simulink model "DegradationParameterMotor"  (R2021a)
settings: Solver=VariableStepAuto  StartTime=0.0  StopTime=10.0  RelTol=1e-3
values from neighbouring files (symbols this model uses):
  mot_P_Fe_Nom_adjustment = 0.5    [Run_GeneratorRectifierBoostConverterInverterMotorModel.m]    (also in Run_InverterMotorModel.m)
  mot_R_s_adjustment = 0.5    [Run_GeneratorRectifierBoostConverterInverterMotorModel.m]    (also in Run_InverterMotorModel.m)
  mot_S_nom_adjustment = 0.5    [Run_GeneratorRectifierBoostConverterInverterMotorModel.m]    (also in Run_InverterMotorModel.m)
undefined symbols (not defined in the file or in its folder): mot_flux_m_adjustment
libraries: Lib_EMTAT x5
settings Model: Creator=sfaulk  LastModifiedBy=mebell

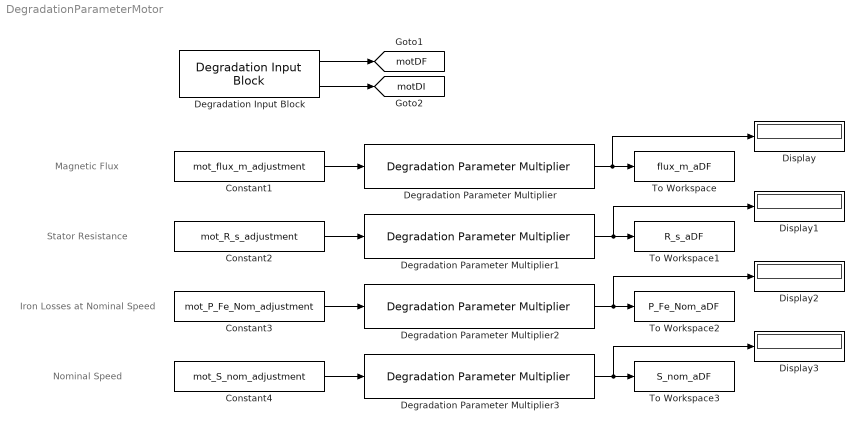
== system DegradationParameterMotor ==
  note: Stator Resistance
  note: Magnetic Flux
  note: Iron Losses at Nominal Speed
  note: Nominal Speed
  Constant1 : Constant  Value=mot_flux_m_adjustment
  Constant2 : Constant  Value=mot_R_s_adjustment
  Constant3 : Constant  Value=mot_P_Fe_Nom_adjustment
  Constant4 : Constant  Value=mot_S_nom_adjustment
  Degradation Input Block : Lib_EMTAT/Components/Physics-Based/Degradation Input Block  SystemSampleTime=-1  VariantActivationTime=update diagram  Latency=0  AutoFrameSizeCalculation=off
      settings: SourceProductName=EMTAT
  Degradation Parameter Multiplier{,1..3} (4 alike) : Lib_EMTAT/Components/Physics-Based/Degradation Parameter Multiplier  SystemSampleTime=-1  VariantActivationTime=update diagram  Latency=0  AutoFrameSizeCalculation=off
      settings: SourceProductName=EMTAT
  Display{,1..3} (4 alike) : Display
  To Workspace : ToWorkspace  VariableName=flux_m_aDF  SaveFormat=Timeseries  SampleTime=-1
      settings: Save2DSignal=2-D array (concatenate along first dimension)
  To Workspace1 : ToWorkspace  VariableName=R_s_aDF  SaveFormat=Timeseries  SampleTime=-1
      settings: Save2DSignal=2-D array (concatenate along first dimension)
  To Workspace2 : ToWorkspace  VariableName=P_Fe_Nom_aDF  SaveFormat=Timeseries  SampleTime=-1
      settings: Save2DSignal=2-D array (concatenate along first dimension)
  To Workspace3 : ToWorkspace  VariableName=S_nom_aDF  SaveFormat=Timeseries  SampleTime=-1
      settings: Save2DSignal=2-D array (concatenate along first dimension)
  tag scope: motDF=global, motDI=global
  wires:
  Constant1/1 -> Degradation Parameter Multiplier/1
  Degradation Parameter Multiplier/1 -> Display/1, To Workspace/1
  Degradation Input Block/2 -> [motDI]
  Degradation Input Block/1 -> [motDF]
  Degradation Parameter Multiplier1/1 -> Display1/1, To Workspace1/1
  Constant2/1 -> Degradation Parameter Multiplier1/1
  Degradation Parameter Multiplier2/1 -> Display2/1, To Workspace2/1
  Constant3/1 -> Degradation Parameter Multiplier2/1
  Constant4/1 -> Degradation Parameter Multiplier3/1
  Degradation Parameter Multiplier3/1 -> Display3/1, To Workspace3/1
